simulink model "Simulation_balanceversionajour2024_avec_statespace"  (R2024a)
settings: Solver=ode4  StartTime=0.0  StopTime=inf  FixedStep=step_time  RelTol=1e-3
InitFcn:
  | Initialisation_simulation
  | beam_build_ss
values from neighbouring files (symbols this model uses):
  A_ss = [zeros(n_modes, n_modes), eye(n_modes) ... (first row only)    [beam_build_ss.m]    (also in lookup_table_statespace.m)
  B_ss = [zeros(n_modes, 1) ... (first row only)    [beam_build_ss.m]    (also in lookup_table_statespace.m)
  C_ss = zeros(2, 2*n_modes)    [beam_build_ss.m]    (also in lookup_table_statespace.m)
  D_ss = zeros(2, 1)    [beam_build_ss.m]    (also in lookup_table_statespace.m)
  denom_com = [R^2*C^2 3*R*C 1]    [Initialisation_simulation.m]
  denom_cou = [1/(2*pi*165) 1]    [Initialisation_simulation.m]
  denom_pos = [1/(2*pi*80) 1]    [Initialisation_simulation.m]
  dL_table = LUT_Table{:,6}    [Initialisation_simulation.m]
  dPhi_table = LUT_Table{:,7}    [Initialisation_simulation.m]
  gain_com = 0.88    [Initialisation_simulation.m]
  gain_cou = 0.716    [Initialisation_simulation.m]
  gain_mod_cou = Gain_Ampli_Puissance(1)    [Initialisation_simulation.m]
  gain_pos = 1.4925    [Initialisation_simulation.m]
  gain_puis = Gain_Ampli_Puissance(1)    [Initialisation_simulation.m]
  kb_table = LUT_Table{:,5}    [Initialisation_simulation.m]
  kd_pos = -0.207    [Initialisation_simulation.m]
  ki_courant = -325    [Initialisation_simulation.m]
  ki_pos = -27.5    [Initialisation_simulation.m]
  kp_courant = -0.575    [Initialisation_simulation.m]
  kp_pos = 2.325    [Initialisation_simulation.m]
  Lb_table = LUT_Table{:,4}    [Initialisation_simulation.m]
  limVampinf = -511.0    (= -511)    [Initialisation_simulation.m]
  limVampmax = 512.0    (= 512)    [Initialisation_simulation.m]
  num_com = 1    [Initialisation_simulation.m]
  num_cou = 1    [Initialisation_simulation.m]
  num_pos = 1    [Initialisation_simulation.m]
  offset_com = -2.5    [Initialisation_simulation.m]
  offset_cou = 3.44    [Initialisation_simulation.m]
  offset_pos = -1.6    [Initialisation_simulation.m]
  per_adc = 1/freq_adc    (= 0.000166666666667)    [Initialisation_simulation.m]
  per_pwm = 1/freq_pwm    (= 6.4e-05)    [Initialisation_simulation.m]
  rb = 1.1745 + 2.349    (= 3.5235)    [Initialisation_simulation.m]
  repos_actionneur = deplacement_statique(idx_force_reduit)    [beam_build_ss.m]    (also in lookup_table_statespace.m = hauteur_encastrement_m + deplacement_statique(idx_force_redu)
  repos_bout = deplacement_statique(idx_bout_reduit)    [beam_build_ss.m]    (also in lookup_table_statespace.m = hauteur_encastrement_m + deplacement_statique(idx_bout_redui)
  sat_com_max = 5    [Initialisation_simulation.m]
  sat_com_min = -5    [Initialisation_simulation.m]
  sat_cou_max = 5    [Initialisation_simulation.m]
  sat_cou_min = 0    [Initialisation_simulation.m]
  sat_pos_max = 5    [Initialisation_simulation.m]
  sat_pos_min = 0    [Initialisation_simulation.m]
  sat_proc_max = 14e-3    (= 0.014)    [Initialisation_simulation.m]    (also in beam_build_ss.m = 1; lookup_table_statespace.m = 1)
  sat_proc_min = 0    [Initialisation_simulation.m]    (also in beam_build_ss.m = -1; lookup_table_statespace.m = -1)
  sat_puis_max = 5    [Initialisation_simulation.m]
  sat_puis_min = -5    [Initialisation_simulation.m]
  SORTIE_POS_MAX = 512.0    (= 512)    [Initialisation_simulation.m]
  SORTIE_POS_MIN = -511.0    (= -511)    [Initialisation_simulation.m]
  step_time = 1/300000    (= 3.33333333333e-06)    [Initialisation_simulation.m]
  Tech = 0.002    [Initialisation_simulation.m]
  Tech_pos = 0.02    [Initialisation_simulation.m]
  tension_selon_distance = polyfit(Distance(1:point_final), Tension(1:point_final), 3)    [Initialisation_simulation.m]
  x_table = LUT_Table{:,2}    [Initialisation_simulation.m]
libraries: simulink_extras x2, simulink x1
settings Model: DataTypeOverride=Double  MinMaxOverflowLogging=ForceOff  Creator=johen30  LastModifiedBy=etmal6

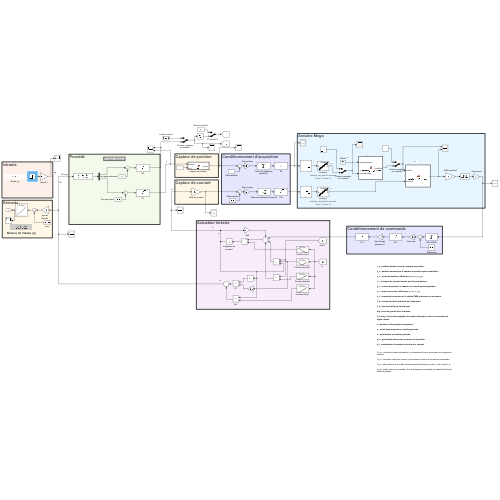
[thumbnail: Simulink's stored preview of the top-level diagram]
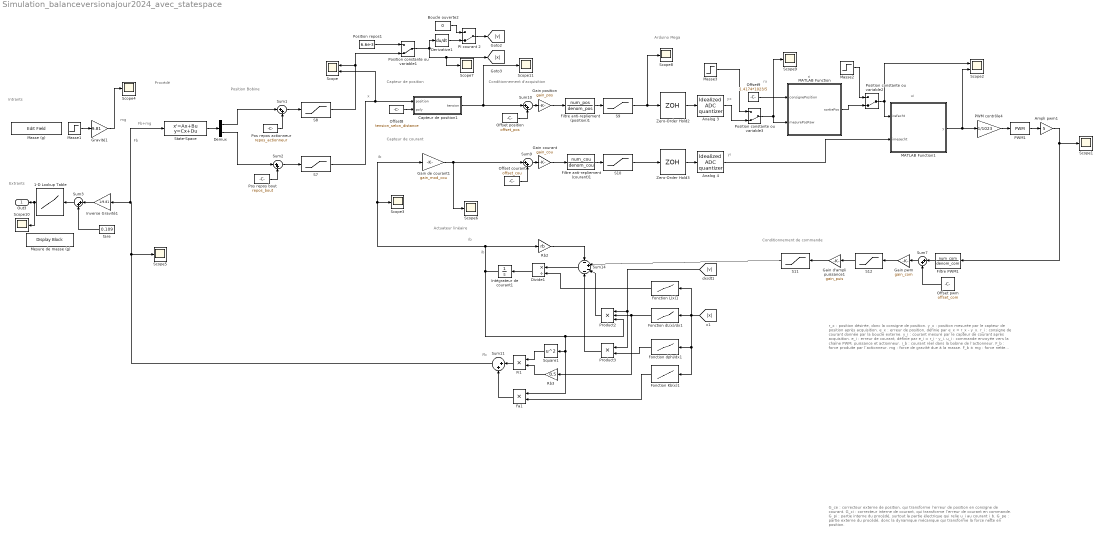
== system Simulation_balanceversionajour2024_avec_statespace ==
  note: ib
  note: x
  note: Capteur de position
  note: Extrants
  note: Conditionnement de commande
  note: Fb
  note: Fb+mg
  note: Position Bobine
  note: ib
  note: Procédé
  note: G_ce : correcteur externe de position, qui transforme l’erreur de position en consigne de courant.
      |
      | G_ci : correcteur interne de courant, qui transforme l’erreur de courant en commande.
      |
      | G_pi : partie interne du procédé, surtout la partie électrique qui relie u_i au courant i_b.
      |
      | G_pe : partie externe du procédé, donc la dynamique mécanique qui transforme la force nette en position.
  note: mg
  note: Capteur de courant
  note: Conditionnement d'acquisition
  note: Arduino Mega
  note: r_x : position désirée, donc la consigne de position.
      |
      | y_x : position mesurée par le capteur de position après acquisition.
      |
      | e_x : erreur de position, définie par e_x = r_x - y_x.
      |
      | r_i : consigne de courant donnée par la boucle externe.
      |
      | y_i : courant mesuré par le capteur de courant après acquisition.
      |
      | e_i : erreur de courant, définie par e_i = r_i - y_i.
      |
      | u_i : commande envoyée vers la chaîne PWM, puissance et actionneur.
      |
      | i_b : courant réel dans la bobine de l’actionneur.
      |
      | F_b : force produite par l’actionneur.
      |
      | mg : force de gravité due à la masse.
      |
      | F_b ± mg : force nette appliquée à la partie mécanique, selon la convention de signe choisie.
      |
      | x : position réelle physique du système.
      |
      | y : sortie finale mesurée en notation générale.
      |
      | d : perturbation en notation générale.
      |
      | d_x : perturbation de mesure ou bruit sur la position.
      |
      | d_i : perturbation de mesure ou bruit sur le courant.
  note: yi
  note: Intrants
  note: rx
  note: yx
  note: ui
  note: ri
  note: Actuateur linéaire
  note: Fb
  note: ib
  1-D Lookup Table : Lookup_n-D  NumberOfTableDimensions=1  BreakpointsForDimension1=[-3.765108647403592e-05, 7.538807411616860e-04, 0.001545188300891, 0.002336345224252, 0.003127396360308, 0.003918370473190, 0.004709286816201, 0.005500158744688, 0.006290995805057, 0.007081804998301, 0.007872591573073]  Table=[0, 10, 20, 30, 40, 50, 60, 70, 80, 90, 100]  InternalRulePriority=Speed  RndMeth=Simplest
  Ampli pwm1 : Gain  Gain=5
  Analog 3 : simulink_extras/Additional Discrete/Idealized ADC quantizer  NumberOfConverterBits=res_adc  Vmin=0  Vmax=5  OutputDataType=int16  OutputNegativeValues=off
  Analog 4 : simulink_extras/Additional Discrete/Idealized ADC quantizer  NumberOfConverterBits=res_adc  Vmin=0  Vmax=5  OutputDataType=int16  OutputNegativeValues=off
  Boucle ouverte2 : Constant  Value=0
  Capteur de position1 : MATLAB Function  TreatAsAtomicUnit=on
  Demux : Demux  Outputs=2
  Derivative1 : Derivative
  Divide1 : Product  Inputs=*/
  Fa1 : Product
  Fi1 : Product
  Filtre PWM1 : TransferFcn  Numerator=num_com  Denominator=denom_com
  Filtre anti-repliement (position)1 : TransferFcn  Numerator=num_pos  Denominator=denom_pos
  Filtre anti-repliement (courant)1 : TransferFcn  Numerator=num_cou  Denominator=denom_cou
  Fonction Kb(x)1 : Lookup_n-D  NumberOfTableDimensions=1  BreakpointsForDimension1=x_table  Table=kb_table  InternalRulePriority=Speed  RndMeth=Simplest
  Fonction L(x)1 : Lookup_n-D  NumberOfTableDimensions=1  BreakpointsForDimension1=x_table  Table=Lb_table  InternalRulePriority=Speed  RndMeth=Simplest
  Fonction dL(x)/dx1 : Lookup_n-D  NumberOfTableDimensions=1  BreakpointsForDimension1=x_table  Table=dL_table  InternalRulePriority=Speed  RndMeth=Simplest
  Fonction dphi/dx1 : Lookup_n-D  NumberOfTableDimensions=1  BreakpointsForDimension1=x_table  Table=dPhi_table  InternalRulePriority=Speed  RndMeth=Simplest
  Gain courant : Gain  Gain=gain_cou
  Gain d'ampli puissance1 : Gain  Gain=gain_puis
  Gain de courant1 : Gain  Gain=gain_mod_cou
  Gain position : Gain  Gain=gain_pos
  Gain pwm : Gain  Gain=gain_com
  Gravité1 : Gain  Gain=9.81
  Intégrateur de courant1 : Integrator
  Inverse Gravité1 : Gain  Gain=1/9.81
  MATLAB Function : MATLAB Function  TreatAsAtomicUnit=on  SystemSampleTime=Tech_pos
  MATLAB Function1 : MATLAB Function  TreatAsAtomicUnit=on  SystemSampleTime=Tech
  Masse (g) : EditField  LabelPosition=Hide  ShowInitialText=on  Alignment=Center
  Masse1 : Step  Time=0  After=61.256  SampleTime=0
  Masse2 : Step  Time=2  After=-100  SampleTime=0
  Masse3 : Step  Time=0.5  After=512  SampleTime=0
  Mesure de masse (g) : DisplayBlock  LabelPosition=Hide  Transparency=1
  Offset courant : Constant  Value=offset_cou
  Offset position : Constant  Value=offset_pos
  Offset pwm : Constant  Value=offset_com
  Offset8 : Constant  Value=tension_selon_distance
  Offset9 : Constant  Value=1.4174*1023/5
  PI courant 2 : ManualSwitch  CurrentSetting=0
  PWM contrôle4 : Gain  Gain=1/1023  OutDataTypeStr=fixdt(1,64, 44)
  PWM1 : simulink/Discontinuities/PWM  DisableCoverage=on  Period=per_pwm  InitialDelay=0  DisallowZeroDutyCycle=off  RunAtFixedTimeIntervals=on  SampleTime=step_time
  Pos repos actionneur : Constant  Value=repos_actionneur
  Pos repos bout : Constant  Value=repos_bout
  Position constante ou variable1 : ManualSwitch  CurrentSetting=0
  Position constante ou variable2 : ManualSwitch  CurrentSetting=0
  Position constante ou variable3 : ManualSwitch  CurrentSetting=0
  Position repos1 : Constant  Value=6.6e-3
  Product2 : Product  Inputs=3
  Product3 : Product
  Rb2 : Gain  Gain=rb
  Rb3 : Gain  Gain=0.5
  S10 : Saturate  UpperLimit=sat_cou_max  LowerLimit=sat_cou_min
  S11 : Saturate  UpperLimit=sat_puis_max  LowerLimit=sat_puis_min
  S12 : Saturate  UpperLimit=sat_com_max  LowerLimit=sat_com_min
  S7 : Saturate  UpperLimit=sat_proc_max  LowerLimit=sat_proc_min  LinearizeAsGain=off
  S8 : Saturate  UpperLimit=sat_proc_max  LowerLimit=sat_proc_min  LinearizeAsGain=off
  S9 : Saturate  UpperLimit=sat_pos_max  LowerLimit=sat_pos_min  LinearizeAsGain=off
  Scope : Scope  NumInputPorts=2
  Scope{1,3..11} (10 alike) : Scope
  Scope2 : Scope  NumInputPorts=2
  Square1 : Math  Operator=square
  State-Space : StateSpace  A=A_ss  B=B_ss  C=C_ss  D=D_ss  InitialCondition=zeros(6,1)
  Sum{1..3,7,9..11} (7 alike) : Sum  Inputs=|++
  Sum14 : Sum  Inputs=-+--
  Zero-Order Hold2 : ZeroOrderHold  SampleTime=per_adc
  Zero-Order Hold3 : ZeroOrderHold  SampleTime=per_adc
  tare : Constant  Value=0.109
  Out3 : Outport
  wires:
  S7/1 -> Scope/2, Capteur de position1/1(position)
  Gain position/1 -> Filtre anti-repliement (position)1/1
  Gain de courant1/1 -> Scope6/1, Sum9/1
  S10/1 -> Zero-Order Hold3/1
  PI courant 2/1 -> [v]
  Gain pwm/1 -> S12/1
  Sum7/1 -> Gain pwm/1
  Derivative1/1 -> PI courant 2/2
  Offset8/1 -> Capteur de position1/2(poly)
  Zero-Order Hold2/1 -> Analog 3/1
  Boucle ouverte2/1 -> PI courant 2/1
  Position repos1/1 -> Position constante ou variable1/1
  Filtre anti-repliement (courant)1/1 -> S10/1
  Ampli pwm1/1 -> Scope1/1, Filtre PWM1/1
  PWM1/1 -> Ampli pwm1/1
  Gravité1/1 -> Scope4/1
  Filtre PWM1/1 -> Sum7/1
  Gain courant/1 -> Filtre anti-repliement (courant)1/1
  Position constante ou variable1/1 -> Derivative1/1, Scope7/1, [x]
  Sum10/1 -> Gain position/1
  Offset position/1 -> Sum10/2
  S8/1 -> Position constante ou variable1/2, Scope/1
  Offset courant/1 -> Sum9/2
  Capteur de position1/1(tension) -> Scope11/1, Sum10/1
  PWM contrôle4/1 -> PWM1/1
  Offset pwm/1 -> Sum7/2
  Sum11/1 -> State-Space/1, Inverse Gravité1/1, Scope5/1
  S12/1 -> Gain d'ampli puissance1/1
  Masse1/1 -> Gravité1/1
  Gain d'ampli puissance1/1 -> S11/1
  Sum9/1 -> Gain courant/1
  Filtre anti-repliement (position)1/1 -> S9/1
  Zero-Order Hold3/1 -> Analog 4/1
  S9/1 -> Scope8/1, Zero-Order Hold2/1
  Analog 4/1 -> MATLAB Function1/2(imesecht)
  MATLAB Function1/1(y) -> Scope2/2, PWM contrôle4/1
  Product2/1 -> Sum14/3
  Fonction Kb(x)1/1 -> Fa1/2
  Divide1/1 -> Intégrateur de courant1/1
  Square1/1 -> Fi1/1
  Intégrateur de courant1/1 -> Scope3/1, Gain de courant1/1, Rb2/1, Fa1/1, Square1/1, Product2/3
  S11/1 -> Sum14/2
  [v] -> Product2/1, Product3/1
  Fa1/1 -> Sum11/2
  Fi1/1 -> Sum11/1
  Fonction dL(x)/dx1/1 -> Rb3/1, Product2/2
  Product3/1 -> Sum14/4
  Fonction L(x)1/1 -> Divide1/2
  Sum14/1 -> Divide1/1
  [x] -> Fonction dL(x)/dx1/1, Fonction L(x)1/1, Fonction dphi/dx1/1, Fonction Kb(x)1/1
  Rb2/1 -> Sum14/1
  Rb3/1 -> Fi1/2
  Fonction dphi/dx1/1 -> Product3/2
  MATLAB Function/1(sortiePos) -> Position constante ou variable2/2
  Position constante ou variable2/1 -> Scope2/1, MATLAB Function1/1(irefecht)
  Masse2/1 -> Position constante ou variable2/1
  Offset9/1 -> MATLAB Function/1(consignePosition)
  Analog 3/1 -> Position constante ou variable3/2
  Masse3/1 -> Position constante ou variable3/1
  Position constante ou variable3/1 -> Scope9/1, MATLAB Function/2(mesurePosRaw)
  State-Space/1 -> Demux/1
  Sum1/1 -> S8/1
  Demux/1 -> Sum1/1
  Demux/2 -> Sum2/1
  Sum2/1 -> S7/1
  Pos repos actionneur/1 -> Sum1/2
  Pos repos bout/1 -> Sum2/2
  tare/1 -> Sum3/2
  Inverse Gravité1/1 -> Sum3/1
  1-D Lookup Table/1 -> Scope10/1, Out3/1
  Sum3/1 -> 1-D Lookup Table/1

== matlab function Simulation_balanceversionajour2024_avec_statespace/Capteur de position1 ==
  data: position input; tension output; poly input
function tension = fct(position, poly)

tension = polyval(poly, position);

== matlab function Simulation_balanceversionajour2024_avec_statespace/MATLAB Function ==
  data: consignePosition input; sortiePos output; mesurePosRaw input; ki_pos parameter; kd_pos parameter; Tech_pos parameter; SORTIE_POS_MIN parameter; SORTIE_POS_MAX parameter; kp_pos parameter
function sortiePos = regulateur_PID_position(consignePosition, mesurePosRaw, ki_pos, kd_pos, Tech_pos, SORTIE_POS_MIN, SORTIE_POS_MAX, kp_pos)
    
    % Constante de temps du filtre dérivé (tirée du code C++ de ton équipe)
    tau_f = 0.09;

    % Calcul des coefficients Tustin à la volée
    den = (2.0 * Tech_pos + 4.0 * tau_f);
    a1 = (4.0 * tau_f) / (Tech_pos + 2.0 * tau_f);
    a2 = (Tech_pos - 2.0 * tau_f) / (Tech_pos + 2.0 * tau_f);

    b0 = (4.0 * kd_pos + ki_pos * Tech_pos^2 + 2.0 * ki_pos * Tech_pos * tau_f + 2.0 * kp_pos * Tech_pos + 4.0 * kp_pos * tau_f) / den;
    b1 = (-8.0 * kd_pos + 2.0 * ki_pos * Tech_pos^2 - 8.0 * kp_pos * tau_f) / den;
    b2 = (4.0 * kd_pos + ki_pos * Tech_pos^2 - 2.0 * ki_pos * Tech_pos * tau_f - 2.0 * kp_pos * Tech_pos + 4.0 * kp_pos * tau_f) / den;

    % Déclaration des variables mémoires (états passés)
    persistent erreurPrecedPos erreurPreced2Pos sortiePrecedPos sortiePreced2Pos;

    % Initialisation au premier appel (t=0)
    if isempty(erreurPrecedPos)
        erreurPrecedPos = 0.0;
        erreurPreced2Pos = 0.0;
        sortiePrecedPos = 0.0;
        sortiePreced2Pos = 0.0;
    end

    % Calcul de l'erreur actuelle
    erreurActuPos = consignePosition - mesurePosRaw;

    % Équation de récurrence (Filtre Tustin)
    sortieBrute = a1 * sortiePrecedPos + ...
                  a2 * sortiePreced2Pos + ...
                  b0 * erreurActuPos + ...
                  b1 * erreurPrecedPos + ...
                  b2 * erreurPreced2Pos;

    % Saturation de la commande de position (Agit aussi comme anti-windup)
    if sortieBrute > SORTIE_POS_MAX
        sortiePos = SORTIE_POS_MAX;
    elseif sortieBrute < SORTIE_POS_MIN
        sortiePos = SORTIE_POS_MIN;
    else
        sortiePos = sortieBrute;
    end

    % Mise à jour des mémoires pour le prochain cycle
    erreurPreced2Pos = erreurPrecedPos;
    erreurPrecedPos  = erreurActuPos;
    sortiePreced2Pos = sortiePrecedPos;
    
    % CRUCIAL : On réinjecte la sortie SATURÉE dans la mémoire
    % C'est ce qui empêche l'intégrale de s'emballer (l'équivalent de l'anti-windup en Tustin)
    sortiePrecedPos  = sortiePos; 

end

== matlab function Simulation_balanceversionajour2024_avec_statespace/MATLAB Function1 ==
  settings: updateMethod=DISCRETE
  data: irefecht input; y output; imesecht input; kp_courant parameter; ki_courant parameter; Tech parameter; limVampinf parameter; limVampmax parameter
function y = regulateur_PI_courant(irefecht, imesecht, kp_courant, ki_courant, Tech, limVampinf, limVampmax)
    % Calcul de l'erreur interne
    errCur = (irefecht + 512) - imesecht;

    % Création de la mémoire pour l'action intégrale
    persistent intCur;
    if isempty(intCur)
        intCur = 0;
    end

    % 1. Mise à jour de l'intégrale (Euler avant)
    intCur = intCur + (errCur * Tech);

    % 2. Calcul du PI brut
    sortieCurUnsat = (kp_courant * errCur) + (ki_courant * intCur);

    % 3. Saturation de la commande (selon tes limites d'entrée)
    if sortieCurUnsat > limVampmax
        sortieCur = limVampmax;
    elseif sortieCurUnsat < limVampinf
        sortieCur = limVampinf;
    else
        sortieCur = sortieCurUnsat;
    end

    % 4. Anti-windup (Empêche l'intégrale de s'emballer si on sature)
    if ((sortieCurUnsat > limVampmax && errCur > 0.0) || ...
        (sortieCurUnsat < limVampinf && errCur < 0.0))
        intCur = intCur - (errCur * Tech);
    end

    % 5. PWM centré (spécifique au code de ton équipe)
    valeurDutyFloat = 512.0 - sortieCur;

    % 6. Saturation finale du PWM (limites matérielles du timer Arduino : 0 à 1023)
    if valeurDutyFloat > 1023.0
        y = 1023.0;
    elseif valeurDutyFloat < 0.0
        y = 0.0;
    else
        y = valeurDutyFloat;
    end
end
